simulink model "projeto_EPLL"  (R2018a)
settings: Solver=ode4  StartTime=0.0  StopTime=1  FixedStep=1e-4  RelTol=1e-3
undefined symbols (not defined in the file): Ibase, L, R, Vdc, Vp
libraries: powerlib_meascontrol x2
settings Model: Creator=lucas.figueiredo  LastModifiedBy=lucas.figueiredo

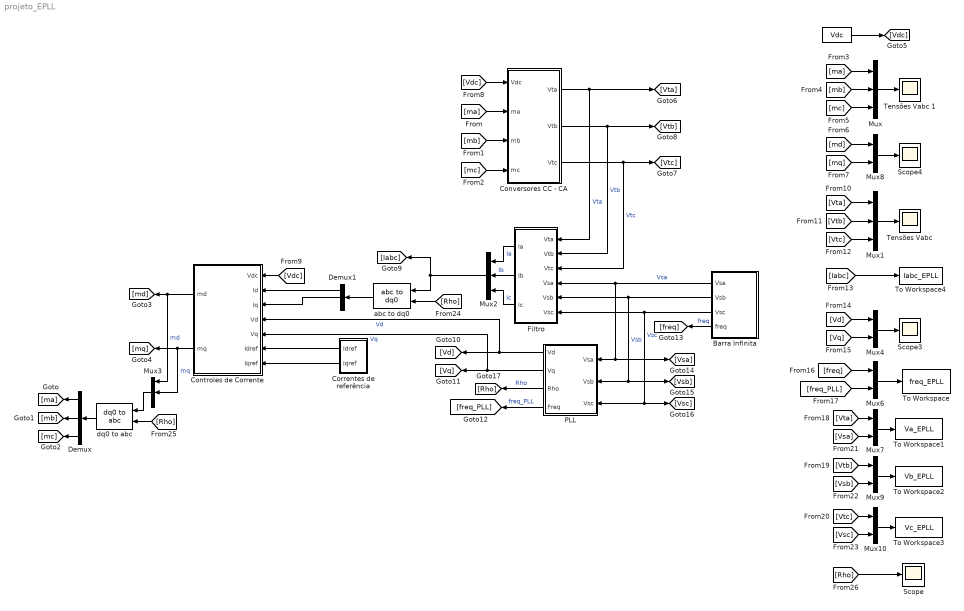
== system projeto_EPLL ==
  " " : Constant  Value=Vdc
  Barra Infinita : Subsystem
  Controles de Corrente : Subsystem
  Conversores CC - CA : Subsystem
  Correntes de referência : Subsystem
  Demux : Demux  Outputs=3
  Demux1 : Demux  Outputs=3
  Filtro : Subsystem
  Mux{,1..3} (4 alike) : Mux  Inputs=3
  Mux{4,6..10} (6 alike) : Mux  Inputs=2
  PLL : Subsystem
  Scope : Scope
  Scope3 : Scope
  Scope4 : Scope
  Tensões Vabc : Scope
  Tensões Vabc 1 : Scope
  To Workspace : ToWorkspace  VariableName=freq_EPLL  SaveFormat=Structure With Time  SampleTime=-1
      settings: Save2DSignal=2-D array (concatenate along first dimension)
  To Workspace1 : ToWorkspace  VariableName=Va_EPLL  SaveFormat=Structure With Time  SampleTime=-1
      settings: Save2DSignal=2-D array (concatenate along first dimension)
  To Workspace2 : ToWorkspace  VariableName=Vb_EPLL  SaveFormat=Structure With Time  SampleTime=-1
      settings: Save2DSignal=2-D array (concatenate along first dimension)
  To Workspace3 : ToWorkspace  VariableName=Vc_EPLL  SaveFormat=Structure With Time  SampleTime=-1
      settings: Save2DSignal=2-D array (concatenate along first dimension)
  To Workspace4 : ToWorkspace  VariableName=Iabc_EPLL  SaveFormat=Structure With Time  SampleTime=-1
      settings: Save2DSignal=2-D array (concatenate along first dimension)
  abc to dq0 : powerlib_meascontrol/Transformations/abc to dq0  Alignment=90 degrees behind phase A axis
  dq0 to abc : powerlib_meascontrol/Transformations/dq0 to abc  Alignment=90 degrees behind phase A axis
  wires:
  Mux/1 -> Tensões Vabc 1/1
  Mux1/1 -> Tensões Vabc/1
  Conversores CC - CA/1(Vta) -> Filtro/1(Vta), [Vta]  "Vta"
  Conversores CC - CA/2(Vtb) -> Filtro/2(Vtb), [Vtb]  "Vtb"
  Conversores CC - CA/3("Vtc ") -> Filtro/3(Vtc), [Vtc]  "Vtc"
  Filtro/1(Ia) -> Mux2/1  "Ia"
  Filtro/2(Ib) -> Mux2/2  "Ib"
  Filtro/3(Ic) -> Mux2/3  "Ic"
  Mux2/1 -> [Iabc], abc to dq0/1
  Mux3/1 -> dq0 to abc/1
  dq0 to abc/1 -> Demux/1
  Barra Infinita/1(Vsa) -> [Vsa], PLL/1(Vsa), Filtro/4(Vsa)  "Vsa"
  Barra Infinita/2(Vsb) -> [Vsb], PLL/2(Vsb), Filtro/5(Vsb)  "Vsb"
  Barra Infinita/3(Vsc) -> [Vsc], PLL/3(Vsc), Filtro/6(Vsc)  "Vsc"
  PLL/1(Vd) -> [Vd], Controles de Corrente/4(Vd)  "Vd"
  PLL/2(Vq) -> [Vq], Controles de Corrente/5(Vq)  "Vq"
  abc to dq0/1 -> Demux1/1
  Demux1/1 -> Controles de Corrente/2(Id)
  Demux1/2 -> Controles de Corrente/3(Iq)
  Controles de Corrente/1(md) -> [md], Mux3/1  "md"
  Controles de Corrente/2(mq) -> [mq], Mux3/2  "mq"
  [ma] -> Conversores CC - CA/2(ma)
  [mb] -> Conversores CC - CA/3(mb)
  [mc] -> Conversores CC - CA/4(mc)
  Demux/1 -> [ma]
  Demux/2 -> [mb]
  Demux/3 -> [mc]
  [ma] -> Mux/1
  [mb] -> Mux/2
  [mc] -> Mux/3
  Mux8/1 -> Scope4/1
  [md] -> Mux8/1
  [mq] -> Mux8/2
  " "/1 -> [Vdc]
  [Vdc] -> Conversores CC - CA/1("Vdc ")
  [Vdc] -> Controles de Corrente/1(Vdc)
  [Vta] -> Mux1/1
  [Vtb] -> Mux1/2
  [Vtc] -> Mux1/3
  [Iabc] -> To Workspace4/1
  Mux4/1 -> Scope3/1
  [Vq] -> Mux4/2
  [Vd] -> Mux4/1
  [freq] -> Mux6/1
  Mux6/1 -> To Workspace/1
  PLL/4(Freq) -> [freq_PLL]  "freq_PLL"
  Barra Infinita/4(freq) -> [freq]  "freq"
  [freq_PLL] -> Mux6/2
  PLL/3(Rho) -> [Rho]  "Rho"
  [Rho] -> abc to dq0/2
  [Rho] -> dq0 to abc/2
  Correntes de referência/1(Idref) -> Controles de Corrente/6(Idref)
  Correntes de referência/2(Iqref) -> Controles de Corrente/7(Iqref)
  [Rho] -> Scope/1
  [Vta] -> Mux7/1
  [Vtc] -> Mux10/1
  [Vsa] -> Mux7/2
  [Vsb] -> Mux9/2
  Mux10/1 -> To Workspace3/1
  Mux9/1 -> To Workspace2/1
  Mux7/1 -> To Workspace1/1
  [Vsc] -> Mux10/2
  [Vtb] -> Mux9/1

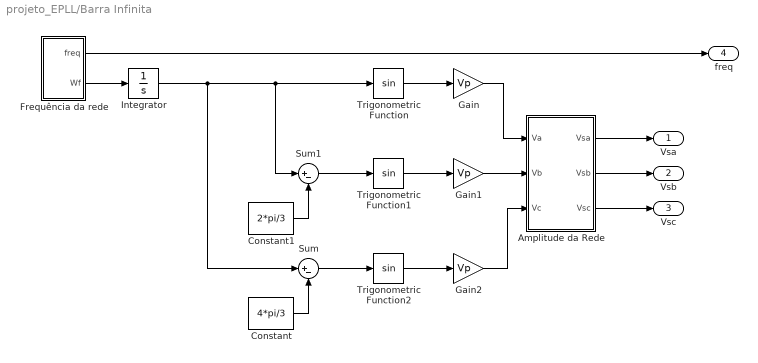
== system projeto_EPLL/Barra Infinita ==
  Amplitude da Rede : Subsystem
  Constant : Constant  Value=4*pi/3
  Constant1 : Constant  Value=2*pi/3
  Frequência da rede : Subsystem
  Gain : Gain  Gain=Vp
  Gain1 : Gain  Gain=Vp
  Gain2 : Gain  Gain=Vp
  Integrator : Integrator
  Sum : Sum  Inputs=|+-
  Sum1 : Sum  Inputs=|+-
  Trigonometric Function : Trigonometry
  Trigonometric Function1 : Trigonometry
  Trigonometric Function2 : Trigonometry
  Vsa : Outport
  Vsb : Outport  Port=2
  Vsc : Outport  Port=3
  freq : Outport  Port=4
  wires:
  Constant1/1 -> Sum1/2
  Frequência da rede/1(freq) -> freq/1
  Trigonometric Function/1 -> Gain/1
  Frequência da rede/2(Wf) -> Integrator/1
  Sum1/1 -> Trigonometric Function1/1
  Gain2/1 -> Amplitude da Rede/3(Vc)
  Constant/1 -> Sum/2
  Trigonometric Function2/1 -> Gain2/1
  Amplitude da Rede/3(Vsc) -> Vsc/1
  Trigonometric Function1/1 -> Gain1/1
  Amplitude da Rede/2(Vsb) -> Vsb/1
  Gain1/1 -> Amplitude da Rede/2(Vb)
  Amplitude da Rede/1(Vsa) -> Vsa/1
  Gain/1 -> Amplitude da Rede/1(Va)
  Sum/1 -> Trigonometric Function2/1
  Integrator/1 -> Sum/1, Sum1/1, Trigonometric Function/1

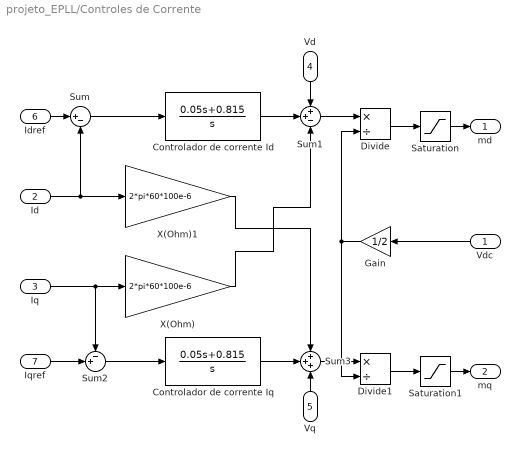
== system projeto_EPLL/Controles de Corrente ==
  Vdc : Inport
  Id : Inport  Port=2
  Iq : Inport  Port=3
  Vd : Inport  Port=4
  Vq : Inport  Port=5
  Idref : Inport  Port=6
  Iqref : Inport  Port=7
  Controlador de corrente Id : TransferFcn  Numerator=[0.05 0.815]  Denominator=[1 0]
  Controlador de corrente Iq : TransferFcn  Numerator=[0.05 0.815]  Denominator=[1 0]
  Divide : Product  Inputs=*/
  Divide1 : Product  Inputs=*/
  Gain : Gain  Gain=1/2
  Saturation : Saturate  UpperLimit=1  LowerLimit=-1
  Saturation1 : Saturate  UpperLimit=1  LowerLimit=-1
  Sum : Sum  Inputs=|+-
  Sum1 : Sum  Inputs=++-
  Sum2 : Sum  Inputs=-+|
  Sum3 : Sum  Inputs=+++
  X(Ohm) : Gain  Gain=2*pi*60*100e-6
  X(Ohm)1 : Gain  Gain=2*pi*60*100e-6
  md : Outport
  mq : Outport  Port=2
  wires:
  Sum2/1 -> Controlador de corrente Iq/1
  Divide1/1 -> Saturation1/1
  Divide/1 -> Saturation/1
  Controlador de corrente Id/1 -> Sum1/2
  Sum3/1 -> Divide1/1
  X(Ohm)1/1 -> Sum3/1
  Iqref/1 -> Sum2/2
  Gain/1 -> Divide1/2, Divide/2
  Controlador de corrente Iq/1 -> Sum3/2
  Sum/1 -> Controlador de corrente Id/1
  Sum1/1 -> Divide/1
  X(Ohm)/1 -> Sum1/3
  Vdc/1 -> Gain/1
  Vq/1 -> Sum3/3
  Vd/1 -> Sum1/1
  Iq/1 -> Sum2/1, X(Ohm)/1
  Id/1 -> Sum/2, X(Ohm)1/1
  Saturation1/1 -> mq/1
  Saturation/1 -> md/1
  Idref/1 -> Sum/1

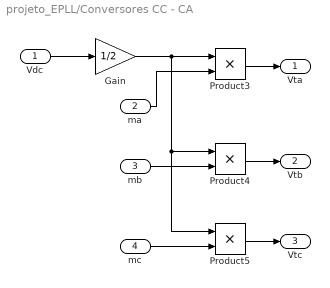
== system projeto_EPLL/Conversores CC - CA ==
  "Vdc " : Inport
  ma : Inport  Port=2
  mb : Inport  Port=3
  mc : Inport  Port=4
  Gain : Gain  Gain=1/2
  Product3 : Product
  Product4 : Product
  Product5 : Product
  Vta : Outport
  Vtb : Outport  Port=2
  "Vtc " : Outport  Port=3
  wires:
  ma/1 -> Product3/2
  mb/1 -> Product4/2
  Product3/1 -> Vta/1
  Gain/1 -> Product4/1, Product5/1, Product3/1
  Product5/1 -> "Vtc "/1
  Product4/1 -> Vtb/1
  "Vdc "/1 -> Gain/1
  mc/1 -> Product5/2

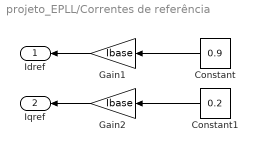
== system projeto_EPLL/Correntes de referência ==
  Constant : Constant  Value=0.9
  Constant1 : Constant  Value=0.2
  Gain1 : Gain  Gain=Ibase
  Gain2 : Gain  Gain=Ibase
  Idref : Outport
  Iqref : Outport  Port=2
  wires:
  Constant1/1 -> Gain2/1
  Constant/1 -> Gain1/1
  Gain2/1 -> Iqref/1
  Gain1/1 -> Idref/1

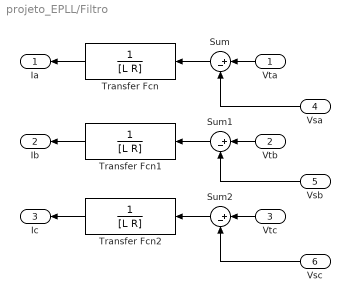
== system projeto_EPLL/Filtro ==
  Vta : Inport
  Vtb : Inport  Port=2
  Vtc : Inport  Port=3
  Vsa : Inport  Port=4
  Vsb : Inport  Port=5
  Vsc : Inport  Port=6
  Sum : Sum  Inputs=|+-
  Sum1 : Sum  Inputs=|+-
  Sum2 : Sum  Inputs=|+-
  Transfer Fcn : TransferFcn  Denominator=[L R]
  Transfer Fcn1 : TransferFcn  Denominator=[L R]
  Transfer Fcn2 : TransferFcn  Denominator=[L R]
  Ia : Outport
  Ib : Outport  Port=2
  Ic : Outport  Port=3
  wires:
  Transfer Fcn1/1 -> Ib/1
  Vtc/1 -> Sum2/1
  Transfer Fcn2/1 -> Ic/1
  Transfer Fcn/1 -> Ia/1
  Sum/1 -> Transfer Fcn/1
  Vta/1 -> Sum/1
  Vsa/1 -> Sum/2
  Sum2/1 -> Transfer Fcn2/1
  Sum1/1 -> Transfer Fcn1/1
  Vtb/1 -> Sum1/1
  Vsc/1 -> Sum2/2
  Vsb/1 -> Sum1/2

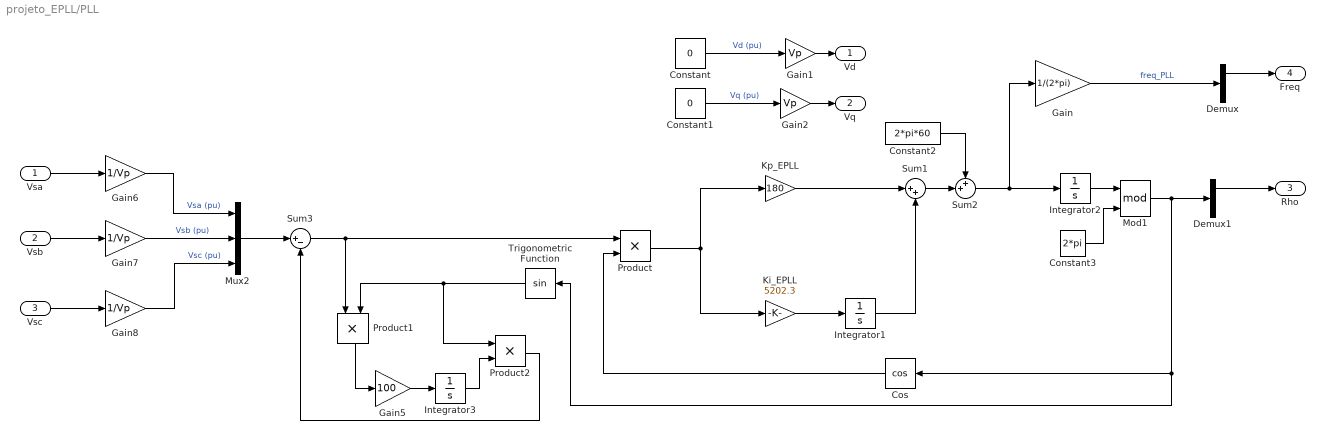
== system projeto_EPLL/PLL ==
  Vsa : Inport
  Vsb : Inport  Port=2
  Vsc : Inport  Port=3
  Constant : Constant  Value=0
  Constant1 : Constant  Value=0
  Constant2 : Constant  Value=2*pi*60
  Constant3 : Constant  Value=2*pi
  Cos : Trigonometry  Operator=cos
  Demux : Demux  Outputs=3
  Demux1 : Demux  Outputs=3
  Gain : Gain  Gain=1/(2*pi)
  Gain1 : Gain  Gain=Vp
  Gain2 : Gain  Gain=Vp
  Gain5 : Gain  Gain=100
  Gain6 : Gain  Gain=1/Vp
  Gain7 : Gain  Gain=1/Vp
  Gain8 : Gain  Gain=1/Vp
  Integrator1 : Integrator
  Integrator2 : Integrator
  Integrator3 : Integrator
  Ki_EPLL : Gain  Gain=5202.3
  Kp_EPLL : Gain  Gain=180
  Mod1 : Math  Operator=mod  SaturateOnIntegerOverflow=on
  Mux2 : Mux  Inputs=3
  Product : Product
  Product1 : Product
  Product2 : Product
  Sum1 : Sum  Inputs=|++
  Sum2 : Sum  Inputs=++|
  Sum3 : Sum  Inputs=|+-
  Trigonometric Function : Trigonometry
  Vd : Outport
  Vq : Outport  Port=2
  Rho : Outport  Port=3
  Freq : Outport  Port=4
  wires:
  Kp_EPLL/1 -> Sum1/1
  Sum2/1 -> Gain/1, Integrator2/1
  Constant2/1 -> Sum2/1
  Constant1/1 -> Gain2/1  "Vq (pu)"
  Constant3/1 -> Mod1/2
  Sum1/1 -> Sum2/2
  Integrator1/1 -> Sum1/2
  Ki_EPLL/1 -> Integrator1/1
  Integrator2/1 -> Mod1/1
  Gain6/1 -> Mux2/1  "Vsa (pu)"
  Vsc/1 -> Gain8/1
  Gain7/1 -> Mux2/2  "Vsb (pu)"
  Gain8/1 -> Mux2/3  "Vsc (pu)"
  Vsb/1 -> Gain7/1
  Vsa/1 -> Gain6/1
  Constant/1 -> Gain1/1  "Vd (pu)"
  Gain1/1 -> Vd/1
  Gain2/1 -> Vq/1
  Product2/1 -> Sum3/2
  Integrator3/1 -> Product2/2
  Gain5/1 -> Integrator3/1
  Mod1/1 -> Demux1/1, Cos/1, Trigonometric Function/1
  Product/1 -> Ki_EPLL/1, Kp_EPLL/1
  Mux2/1 -> Sum3/1
  Trigonometric Function/1 -> Product2/1, Product1/2
  Sum3/1 -> Product1/1, Product/1
  Cos/1 -> Product/2
  Product1/1 -> Gain5/1
  Gain/1 -> Demux/1  "freq_PLL"
  Demux/1 -> Freq/1
  Demux1/1 -> Rho/1

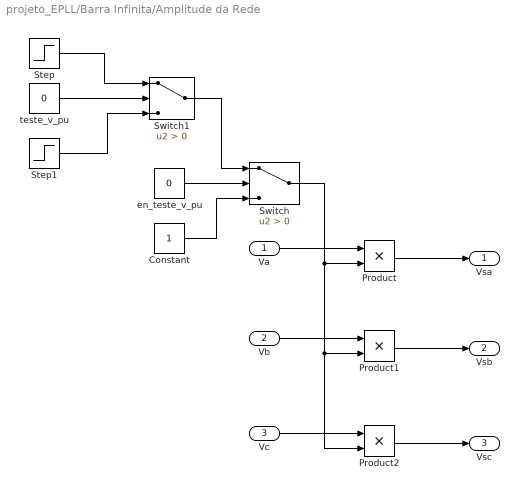
== system projeto_EPLL/Barra Infinita/Amplitude da Rede ==
  Va : Inport
  Vb : Inport  Port=2
  Vc : Inport  Port=3
  Constant : Constant
  Product : Product
  Product1 : Product
  Product2 : Product
  Step : Step  Time=0.3  Before=1  After=1.1  SampleTime=0
  Step1 : Step  Time=0.3  Before=1  After=0.9  SampleTime=0
  Switch : Switch  Criteria=u2 > Threshold
  Switch1 : Switch  Criteria=u2 > Threshold
  en_teste_v_pu : Constant  Value=0
  teste_v_pu : Constant  Value=0
  Vsa : Outport
  Vsb : Outport  Port=2
  Vsc : Outport  Port=3
  wires:
  Product/1 -> Vsa/1
  Switch/1 -> Product/2, Product1/2, Product2/2
  Vb/1 -> Product1/1
  Vc/1 -> Product2/1
  Va/1 -> Product/1
  Product2/1 -> Vsc/1
  Product1/1 -> Vsb/1
  en_teste_v_pu/1 -> Switch/2
  Constant/1 -> Switch/3
  Switch1/1 -> Switch/1
  teste_v_pu/1 -> Switch1/2
  Step/1 -> Switch1/1
  Step1/1 -> Switch1/3

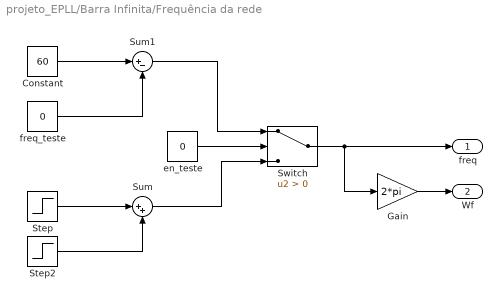
== system projeto_EPLL/Barra Infinita/Frequência da rede ==
  Constant : Constant  Value=60
  Gain : Gain  Gain=2*pi
  Step : Step  Time=0.2  Before=60  After=50  SampleTime=0
  Step2 : Step  Time=0.4  After=10  SampleTime=0
  Sum : Sum  Inputs=|++
  Sum1 : Sum  Inputs=|+-
  Switch : Switch  Criteria=u2 > Threshold
  en_teste : Constant  Value=0
  freq_teste : Constant  Value=0
  freq : Outport
  Wf : Outport  Port=2
  wires:
  Gain/1 -> Wf/1
  Switch/1 -> Gain/1, freq/1
  Step/1 -> Sum/1
  Step2/1 -> Sum/2
  en_teste/1 -> Switch/2
  freq_teste/1 -> Sum1/2
  Constant/1 -> Sum1/1
  Sum/1 -> Switch/3
  Sum1/1 -> Switch/1
